simulink model "souk_single_pipeline_krm"  (R2021a)
settings: Solver=VariableStepAuto  StartTime=0.0  StopTime=10.0  RelTol=1e-3
undefined symbols (not defined in the file): datetime, emio_enet2_tsu_timer_cmp_val_0, posixtime, signal
libraries: xbsIndex_r4 x9043, casper_library_misc x75, casper_library_delays x33, casper_library_reorder x22, xps_library x11
(part 12 of 101)

== system souk_single_pipeline_krm/p0/synth_input_reorder ==
  note: split even / odd channels to separate streams,
      | since the downstream OS synth bank operates
      | on even and odd channels with independent
      | PSBs
  note: And now reverse back to multiple channels
      | per word
  sync : Inport
  din : Inport  Port=2
  rst : Inport  Port=3
  3 : Subsystem  AncestorBlock=casper_library_reorder/reorder  mask(reorder){map=reshape(transpose(reshape([0:2^(serial_chan_bits + parallel_samp_bits)-1], 2^parallel_samp_bits, [])), 2^(serial_chan_bits + parallel_samp_bits), []), n_bits=0, n_inputs=1, bram_latency=2, map_latency=1, fanout_latency=0, double_buffer=1, bram_map=off, software_controlled=off, use_control_fanout=on, hide_latency=on}
      mask prompts: map "Output Order:"; n_bits "Data width in"; n_inputs "Number of inputs"; bram_latency "BRAM Latency"; map_latency "Map Latency"; fanout_latency "Fanout latency"; double_buffer "Double Buffer"; bram_map "Use BlockRAM for Map"; software_controlled "Use runtime software control"; use_control_fanout "Control fanout of control to multiple iniputs"; hide_latency "EXPERIMENTAL: Hide control latency"
      mask init: same as souk_single_pipeline_krm/p0/chan_select/2
      settings: AttributesFormatString=order=2
      mask Help: eval('xlWeb(''http://casper.berkeley.edu/wiki/Reorder'')')
  Constant : xbsIndex_r4/Constant  Commented=on  const=1.0  gui_display_data_type=Boolean  arith_type=Boolean  n_bits=16  bin_pt=14  preci_type=Single  exp_width=8  frac_width=24  explicit_period=on  period=1  equ=P=C  opselect=C  inp2=PCIN>>17  opr=+  inp1=P  carry=CIN  dbl_ovrd=off  block_type=constant
  Constant4 : xbsIndex_r4/Constant  const=1.0  gui_display_data_type=Boolean  arith_type=Boolean  n_bits=16  bin_pt=14  preci_type=Single  exp_width=8  frac_width=24  explicit_period=on  period=1  equ=P=C  opselect=C  inp2=PCIN>>17  opr=+  inp1=P  carry=CIN  dbl_ovrd=off  block_type=constant
  Constant6 : xbsIndex_r4/Constant  Commented=on  const=2^15 - 1  gui_display_data_type=Fixed-point  arith_type=Unsigned  n_bits=15  bin_pt=0  preci_type=Single  exp_width=8  frac_width=24  explicit_period=on  period=1  equ=P=C  opselect=C  inp2=PCIN>>17  opr=+  inp1=P  carry=CIN  dbl_ovrd=off  block_type=constant
  Constant7 : xbsIndex_r4/Constant  Commented=on  const=1.0  gui_display_data_type=Boolean  arith_type=Boolean  n_bits=16  bin_pt=14  preci_type=Single  exp_width=8  frac_width=24  explicit_period=on  period=1  equ=P=C  opselect=C  inp2=PCIN>>17  opr=+  inp1=P  carry=CIN  dbl_ovrd=off  block_type=constant
  Counter : xbsIndex_r4/Counter  Commented=on  cnt_type=Free Running  cnt_to=Inf  operation=Up  start_count=0  cnt_by_val=1  arith_type=Unsigned  n_bits=15  bin_pt=0  load_pin=off  rst=on  en=off  explicit_period=on  period=1  use_behavioral_HDL=off  implementation=Fabric  dbl_ovrd=off  block_type=counter
  Delay1 : xbsIndex_r4/Delay  rst=off  infoeditControl=Selection of Reset will increase slice count due to use of real FFs and instead of SRLs  en=off  latency=0  reg_retiming=on  dbl_ovrd=off  block_type=delay
  Relational : xbsIndex_r4/Relational  Commented=on  mode=a=b  op_type=Bool  en=off  latency=0  dbl_ovrd=off  block_type=relational
  bus_convert : Subsystem  Commented=on  AncestorBlock=casper_library_bus/bus_convert  mask(bus_convert){n_bits_in=ones(8,1) * 18, bin_pt_in=17, cmplx=on, n_bits_out=16, bin_pt_out=15, quantization=0, overflow=0, csp_latency=0, of=off, misc=off}
      mask prompts: n_bits_in "input bit widths"; bin_pt_in "input binary points"; cmplx "input complex"; n_bits_out "output bit widths"; bin_pt_out "output binary points"; quantization "quantization strategy (Truncate=0, Round  (unbiased: +/- Inf)=1, Round (unbiased: Even Values)=2)"; overflow "overflow strategy (Wrap=0, Saturate=1, Flag as error=2)"; csp_latency "latency"; of "overflow indication"; misc "misc support"
      mask help: Convert components of busses
      mask init: same as souk_single_pipeline_krm/common/cordic_gen/bus_convert
  bus_convert1 : Subsystem  Commented=on  AncestorBlock=casper_library_bus/bus_convert  mask(bus_convert){n_bits_in=ones(8,1) * 18, bin_pt_in=17, cmplx=on, n_bits_out=16, bin_pt_out=15, quantization=0, overflow=0, csp_latency=0, of=off, misc=off}
      mask prompts: n_bits_in "input bit widths"; bin_pt_in "input binary points"; cmplx "input complex"; n_bits_out "output bit widths"; bin_pt_out "output binary points"; quantization "quantization strategy (Truncate=0, Round  (unbiased: +/- Inf)=1, Round (unbiased: Even Values)=2)"; overflow "overflow strategy (Wrap=0, Saturate=1, Flag as error=2)"; csp_latency "latency"; of "overflow indication"; misc "misc support"
      mask help: Convert components of busses
      mask init: same as souk_single_pipeline_krm/common/cordic_gen/bus_convert
  bus_convert2 : Subsystem  AncestorBlock=casper_library_bus/bus_convert  mask(bus_convert){n_bits_in=ones(4,1)*24, bin_pt_in=22, cmplx=on, n_bits_out=18, bin_pt_out=17, quantization=2, overflow=1, csp_latency=0, of=off, misc=off}
      mask prompts: n_bits_in "input bit widths"; bin_pt_in "input binary points"; cmplx "input complex"; n_bits_out "output bit widths"; bin_pt_out "output binary points"; quantization "quantization strategy (Truncate=0, Round  (unbiased: +/- Inf)=1, Round (unbiased: Even Values)=2)"; overflow "overflow strategy (Wrap=0, Saturate=1, Flag as error=2)"; csp_latency "latency"; of "overflow indication"; misc "misc support"
      mask help: Convert components of busses
      mask init: same as souk_single_pipeline_krm/common/cordic_gen/bus_convert
  bus_create : Subsystem  AncestorBlock=casper_library_flow_control/bus_create  mask(bus_create){inputNum=2^(parallel_chan_bits - parallel_samp_bits)}
      mask prompts: inputNum "Number of inputs:"
      mask init:
      | bus_create_init(gcb,...
      |     'inputNum', inputNum);
  bus_create1 : Subsystem  AncestorBlock=casper_library_flow_control/bus_create  mask(bus_create){inputNum=2^(parallel_samp_bits)}
      mask prompts: inputNum "Number of inputs:"
      mask init:
      | bus_create_init(gcb,...
      |     'inputNum', inputNum);
  bus_create2 : Subsystem  AncestorBlock=casper_library_flow_control/bus_create  mask(bus_create){inputNum=2^(parallel_samp_bits)}
      mask prompts: inputNum "Number of inputs:"
      mask init:
      | bus_create_init(gcb,...
      |     'inputNum', inputNum);
  bus_create3 : Subsystem  AncestorBlock=casper_library_flow_control/bus_create  mask(bus_create){inputNum=2^(parallel_samp_bits)}
      mask prompts: inputNum "Number of inputs:"
      mask init:
      | bus_create_init(gcb,...
      |     'inputNum', inputNum);
  bus_create4 : Subsystem  AncestorBlock=casper_library_flow_control/bus_create  mask(bus_create){inputNum=2^(parallel_samp_bits)}
      mask prompts: inputNum "Number of inputs:"
      mask init:
      | bus_create_init(gcb,...
      |     'inputNum', inputNum);
  bus_expand : Subsystem  AncestorBlock=casper_library_flow_control/bus_expand  mask(bus_expand){mode=divisions of equal size, outputNum=2, outputWidth=36 * 2^(parallel_chan_bits-1), outputBinaryPt=0, outputArithmeticType=0, show_format=off, outputToWorkspace=off, variablePrefix=out, outputToModelAsWell=on}
      mask prompts: outputNum "Number of outputs:"; outputWidth "Output width:"; outputBinaryPt "Output binary point position:"; outputArithmeticType "Output arithmetic type (ufix=0, fix=1, bool=2):"; show_format "Print format string?"; outputToWorkspace "Output to workspace?"; variablePrefix "Variable name prefix:"; outputToModelAsWell "Output to model as well?"
      mask help:
      | Expands a 'bus' made using a bus_create or Xilinx
      | concat block.
      | The input will be divided into the specified number
      | of outputs with the specified arithmetic types.
      | Divisions are made from most significant bit.
      mask init: same as souk_single_pipeline_krm/bus_expand
      settings: AttributesFormatString=2 outputs
      mask TypeOptions mode: divisions of equal size | divisions of arbitrary size
      mask Callback mode: %bus_expand_callback();
      mask Callback outputWidth: %bus_expand_callback();
      mask Callback outputToWorkspace: %bus_expand_callback();
  bus_expand1 : Subsystem  AncestorBlock=casper_library_flow_control/bus_expand  mask(bus_expand){mode=divisions of equal size, outputNum=2^parallel_samp_bits, outputWidth=18*2, outputBinaryPt=0, outputArithmeticType=0, show_format=off, outputToWorkspace=off, variablePrefix=out, outputToModelAsWell=on}
      mask prompts: outputNum "Number of outputs:"; outputWidth "Output width:"; outputBinaryPt "Output binary point position:"; outputArithmeticType "Output arithmetic type (ufix=0, fix=1, bool=2):"; show_format "Print format string?"; outputToWorkspace "Output to workspace?"; variablePrefix "Variable name prefix:"; outputToModelAsWell "Output to model as well?"
      mask help:
      | Expands a 'bus' made using a bus_create or Xilinx
      | concat block.
      | The input will be divided into the specified number
      | of outputs with the specified arithmetic types.
      | Divisions are made from most significant bit.
      mask init: same as souk_single_pipeline_krm/bus_expand
      settings: AttributesFormatString=4 outputs
      mask TypeOptions mode: divisions of equal size | divisions of arbitrary size
      mask Callback mode: %bus_expand_callback();
      mask Callback outputWidth: %bus_expand_callback();
      mask Callback outputToWorkspace: %bus_expand_callback();
  bus_expand2 : Subsystem  AncestorBlock=casper_library_flow_control/bus_expand  mask(bus_expand){mode=divisions of equal size, outputNum=2^parallel_samp_bits, outputWidth=18*2, outputBinaryPt=0, outputArithmeticType=0, show_format=off, outputToWorkspace=off, variablePrefix=out, outputToModelAsWell=on}
      mask prompts: outputNum "Number of outputs:"; outputWidth "Output width:"; outputBinaryPt "Output binary point position:"; outputArithmeticType "Output arithmetic type (ufix=0, fix=1, bool=2):"; show_format "Print format string?"; outputToWorkspace "Output to workspace?"; variablePrefix "Variable name prefix:"; outputToModelAsWell "Output to model as well?"
      mask help:
      | Expands a 'bus' made using a bus_create or Xilinx
      | concat block.
      | The input will be divided into the specified number
      | of outputs with the specified arithmetic types.
      | Divisions are made from most significant bit.
      mask init: same as souk_single_pipeline_krm/bus_expand
      settings: AttributesFormatString=4 outputs
      mask TypeOptions mode: divisions of equal size | divisions of arbitrary size
      mask Callback mode: %bus_expand_callback();
      mask Callback outputWidth: %bus_expand_callback();
      mask Callback outputToWorkspace: %bus_expand_callback();
  bus_expand3 : Subsystem  AncestorBlock=casper_library_flow_control/bus_expand  mask(bus_expand){mode=divisions of equal size, outputNum=2^parallel_samp_bits, outputWidth=18*2, outputBinaryPt=0, outputArithmeticType=0, show_format=off, outputToWorkspace=off, variablePrefix=out, outputToModelAsWell=on}
      mask prompts: outputNum "Number of outputs:"; outputWidth "Output width:"; outputBinaryPt "Output binary point position:"; outputArithmeticType "Output arithmetic type (ufix=0, fix=1, bool=2):"; show_format "Print format string?"; outputToWorkspace "Output to workspace?"; variablePrefix "Variable name prefix:"; outputToModelAsWell "Output to model as well?"
      mask help:
      | Expands a 'bus' made using a bus_create or Xilinx
      | concat block.
      | The input will be divided into the specified number
      | of outputs with the specified arithmetic types.
      | Divisions are made from most significant bit.
      mask init: same as souk_single_pipeline_krm/bus_expand
      settings: AttributesFormatString=4 outputs
      mask TypeOptions mode: divisions of equal size | divisions of arbitrary size
      mask Callback mode: %bus_expand_callback();
      mask Callback outputWidth: %bus_expand_callback();
      mask Callback outputToWorkspace: %bus_expand_callback();
  bus_expand4 : Subsystem  AncestorBlock=casper_library_flow_control/bus_expand  mask(bus_expand){mode=divisions of equal size, outputNum=2^parallel_samp_bits, outputWidth=18*2, outputBinaryPt=0, outputArithmeticType=0, show_format=off, outputToWorkspace=off, variablePrefix=out, outputToModelAsWell=on}
      mask prompts: outputNum "Number of outputs:"; outputWidth "Output width:"; outputBinaryPt "Output binary point position:"; outputArithmeticType "Output arithmetic type (ufix=0, fix=1, bool=2):"; show_format "Print format string?"; outputToWorkspace "Output to workspace?"; variablePrefix "Variable name prefix:"; outputToModelAsWell "Output to model as well?"
      mask help:
      | Expands a 'bus' made using a bus_create or Xilinx
      | concat block.
      | The input will be divided into the specified number
      | of outputs with the specified arithmetic types.
      | Divisions are made from most significant bit.
      mask init: same as souk_single_pipeline_krm/bus_expand
      settings: AttributesFormatString=4 outputs
      mask TypeOptions mode: divisions of equal size | divisions of arbitrary size
      mask Callback mode: %bus_expand_callback();
      mask Callback outputWidth: %bus_expand_callback();
      mask Callback outputToWorkspace: %bus_expand_callback();
  map0 : Subsystem  mask{vec_len_bits=11, ram_latency=2, sample_width=18, n_samples=2^parallel_samp_bits, add_latency=2}
      mask prompts: vec_len_bits "Vector length (2^?)"; ram_latency "Ram Latency"; sample_width "data width per sample"; n_samples "Number of samples per word"; add_latency "Adder latency"
  map1 : Subsystem  mask{vec_len_bits=11, ram_latency=2, sample_width=18, n_samples=2^parallel_samp_bits, add_latency=2}
      mask prompts: vec_len_bits "Vector length (2^?)"; ram_latency "Ram Latency"; sample_width "data width per sample"; n_samples "Number of samples per word"; add_latency "Adder latency"
  map2 : Subsystem  mask{vec_len_bits=11, ram_latency=2, sample_width=18, n_samples=2^parallel_samp_bits, add_latency=2}
      mask prompts: vec_len_bits "Vector length (2^?)"; ram_latency "Ram Latency"; sample_width "data width per sample"; n_samples "Number of samples per word"; add_latency "Adder latency"
  map3 : Subsystem  mask{vec_len_bits=11, ram_latency=2, sample_width=18, n_samples=2^parallel_samp_bits, add_latency=2}
      mask prompts: vec_len_bits "Vector length (2^?)"; ram_latency "Ram Latency"; sample_width "data width per sample"; n_samples "Number of samples per word"; add_latency "Adder latency"
  munge1 : Subsystem  AncestorBlock=casper_library_flow_control/munge  mask(munge){divisions=2^parallel_chan_bits, div_size=ones(2^parallel_chan_bits, 1) * 36, order=reshape(transpose(reshape([0:2^parallel_chan_bits - 1], 2, [])), 1, []), arith_type_out=Unsigned, bin_pt_out=0}
      mask prompts: divisions "Number of divisions"; div_size "Division size (bits)"; order "Division packing order"; arith_type_out "Output arithmetic type"; bin_pt_out "Output binary point"
      mask help: Splits an input bus into the specified number of divisions and then recombines them in the order specified (most significant division = 0,least = number divisions-1)
      mask init:
      | munge_init(gcb, ...
      |     'divisions', divisions, ...
      |     'div_size', div_size, ...
      |     'order', order, ...
      |     'arith_type_out', arith_type_out, ...
      |     'bin_pt_out', bin_pt_out);
      settings: AttributesFormatString=|
      | split:[36;36;36;36;36;36;36;36;36;36;36;36;36;36;36;36]
      | join:[0 2 4 6 8 10 12 14 1 3 5 7 9 11 13 15]
      | Unsigned [576,0]
      mask TypeOptions arith_type_out: Unsigned | Signed  (2's comp) | Floating-point
  snapshot0 : Subsystem  Tag=casper:snapshot  Commented=on  AncestorBlock=casper_library_scopes/snapshot  mask(snapshot){storage=bram, dram_dimm=2, dram_clock=250, nsamples=13, data_width=256, offset=off, circap=off, value=off, ext_arm=off, ext_circ=off, provide_outputs=on, use_dsp48=off}
      mask prompts: storage "Storage medium"; dram_dimm "DRAM dimm"; dram_clock "DRAM clock rate"; nsamples "Number of Samples (2^?)"; data_width "Data width"; offset "Start delay support"; circap "Circular capture support"; value "Extra value capture support"; ext_arm "External arm support"; ext_circ "External circular capture support"; provide_outputs "Provide outputs"; use_dsp48 "Use DSP48s to implement counters"
      mask help:
      | Standard snap block, but with the following optional extras;
      |  1) Optionally delay the fabric trigger by a user-specified number of valids.
      |  2) Capture continuously after a trigger until a stop pulse is received. Data is captured into BRAM continuously, with old data being overwritten until a stop command is received. Then stop capturing when memory is filled. This enables you to get some data before and some data after the stop pulse. Use the 'tr_en_cnt' register to determine where you are in your vector. 'Addr' register's MSb now indicates 'busy capturing'.
      |  3) Optionally capture a value on an input port to a register at the same time as the first data sample.
      |  4) Implement counters using DSP48Es to save resources.
      mask init: same as souk_single_pipeline_krm/p0/acc0/snapshot
      settings: AttributesFormatString=|
      | 256 wide, 8192 deep
      | debugID: 87241941
      mask TypeOptions storage: bram | dram
      mask Callback storage: snapshot_callback();
      mask TypeOptions dram_dimm: 1 | 2 | 3 | 4
      mask TypeOptions dram_clock: 200 | 250 | 266 | 300 | 333
      mask TypeOptions data_width: 8 | 16 | 32 | 64 | 128 | 256 | 512 | 1024
  snapshot1 : Subsystem  Tag=casper:snapshot  Commented=on  AncestorBlock=casper_library_scopes/snapshot  mask(snapshot){storage=bram, dram_dimm=2, dram_clock=250, nsamples=13, data_width=256, offset=off, circap=off, value=off, ext_arm=off, ext_circ=off, provide_outputs=on, use_dsp48=off}
      mask prompts: storage "Storage medium"; dram_dimm "DRAM dimm"; dram_clock "DRAM clock rate"; nsamples "Number of Samples (2^?)"; data_width "Data width"; offset "Start delay support"; circap "Circular capture support"; value "Extra value capture support"; ext_arm "External arm support"; ext_circ "External circular capture support"; provide_outputs "Provide outputs"; use_dsp48 "Use DSP48s to implement counters"
      mask help:
      | Standard snap block, but with the following optional extras;
      |  1) Optionally delay the fabric trigger by a user-specified number of valids.
      |  2) Capture continuously after a trigger until a stop pulse is received. Data is captured into BRAM continuously, with old data being overwritten until a stop command is received. Then stop capturing when memory is filled. This enables you to get some data before and some data after the stop pulse. Use the 'tr_en_cnt' register to determine where you are in your vector. 'Addr' register's MSb now indicates 'busy capturing'.
      |  3) Optionally capture a value on an input port to a register at the same time as the first data sample.
      |  4) Implement counters using DSP48Es to save resources.
      mask init: same as souk_single_pipeline_krm/p0/acc0/snapshot
      settings: AttributesFormatString=|
      | 256 wide, 8192 deep
      | debugID: 87241941
      mask TypeOptions storage: bram | dram
      mask Callback storage: snapshot_callback();
      mask TypeOptions dram_dimm: 1 | 2 | 3 | 4
      mask TypeOptions dram_clock: 200 | 250 | 266 | 300 | 333
      mask TypeOptions data_width: 8 | 16 | 32 | 64 | 128 | 256 | 512 | 1024
  square_transposer1 : Subsystem  AncestorBlock=casper_library_reorder/square_transposer  mask(square_transposer){n_inputs=parallel_samp_bits, async=off}
      mask prompts: n_inputs "Number of inputs (2^?):"; async "Aynchronus operation"
      mask init:
      | square_transposer_init(gcb,...
      |     'n_inputs', n_inputs, ...
      |     'async', async);
      settings: AttributesFormatString=n_inputs=2
      mask Help: eval('xlWeb(''http://casper.berkeley.edu/wiki/Square_transposer'')')
  square_transposer2 : Subsystem  AncestorBlock=casper_library_reorder/square_transposer  mask(square_transposer){n_inputs=parallel_samp_bits, async=off}
      mask prompts: n_inputs "Number of inputs (2^?):"; async "Aynchronus operation"
      mask init:
      | square_transposer_init(gcb,...
      |     'n_inputs', n_inputs, ...
      |     'async', async);
      settings: AttributesFormatString=n_inputs=2
      mask Help: eval('xlWeb(''http://casper.berkeley.edu/wiki/Square_transposer'')')
  square_transposer3 : Subsystem  AncestorBlock=casper_library_reorder/square_transposer  mask(square_transposer){n_inputs=parallel_samp_bits, async=off}
      mask prompts: n_inputs "Number of inputs (2^?):"; async "Aynchronus operation"
      mask init:
      | square_transposer_init(gcb,...
      |     'n_inputs', n_inputs, ...
      |     'async', async);
      settings: AttributesFormatString=n_inputs=2
      mask Help: eval('xlWeb(''http://casper.berkeley.edu/wiki/Square_transposer'')')
  square_transposer4 : Subsystem  AncestorBlock=casper_library_reorder/square_transposer  mask(square_transposer){n_inputs=parallel_samp_bits, async=off}
      mask prompts: n_inputs "Number of inputs (2^?):"; async "Aynchronus operation"
      mask init:
      | square_transposer_init(gcb,...
      |     'n_inputs', n_inputs, ...
      |     'async', async);
      settings: AttributesFormatString=n_inputs=2
      mask Help: eval('xlWeb(''http://casper.berkeley.edu/wiki/Square_transposer'')')
  sync_out : Outport  VectorParamsAs1DForOutWhenUnconnected=off
  dout0 : Outport  Port=2  VectorParamsAs1DForOutWhenUnconnected=off
  dout1 : Outport  Port=3  VectorParamsAs1DForOutWhenUnconnected=off
  wires:
  bus_create4/1(bus_out) -> bus_create/4(in4)
  bus_create1/1(bus_out) -> bus_create/1(in1)
  bus_create3/1(bus_out) -> bus_create/3(in3)
  bus_create2/1(bus_out) -> bus_create/2(in2)
  map3/1(sync_out) -> square_transposer4/1(sync)
  map3/2(dout) -> bus_expand4/1(bus_in)
  square_transposer4/2(out0) -> bus_create4/1(in1)
  square_transposer4/3(out1) -> bus_create4/2(in2)
  square_transposer4/4(out2) -> bus_create4/3(in3)
  square_transposer4/5(out3) -> bus_create4/4(in4)
  bus_expand4/1(msb_out4) -> square_transposer4/2(in0)
  bus_expand4/2(out3) -> square_transposer4/3(in1)
  bus_expand4/3(out2) -> square_transposer4/4(in2)
  bus_expand4/4(lsb_out1) -> square_transposer4/5(in3)
  bus_expand3/4(lsb_out1) -> square_transposer3/5(in3)
  bus_expand3/3(out2) -> square_transposer3/4(in2)
  bus_expand3/2(out3) -> square_transposer3/3(in1)
  bus_expand3/1(msb_out4) -> square_transposer3/2(in0)
  square_transposer3/5(out3) -> bus_create3/4(in4)
  square_transposer3/4(out2) -> bus_create3/3(in3)
  square_transposer3/3(out1) -> bus_create3/2(in2)
  square_transposer3/2(out0) -> bus_create3/1(in1)
  map2/2(dout) -> bus_expand3/1(bus_in)
  map2/1(sync_out) -> square_transposer3/1(sync)
  map1/1(sync_out) -> square_transposer2/1(sync)
  map1/2(dout) -> bus_expand2/1(bus_in)
  square_transposer2/2(out0) -> bus_create2/1(in1)
  square_transposer2/3(out1) -> bus_create2/2(in2)
  square_transposer2/4(out2) -> bus_create2/3(in3)
  square_transposer2/5(out3) -> bus_create2/4(in4)
  bus_expand2/1(msb_out4) -> square_transposer2/2(in0)
  bus_expand2/2(out3) -> square_transposer2/3(in1)
  bus_expand2/3(out2) -> square_transposer2/4(in2)
  bus_expand2/4(lsb_out1) -> square_transposer2/5(in3)
  bus_create/1(bus_out) -> 3/3(din0)
  munge1/1(dout) -> bus_expand/1(bus_in)
  bus_expand/1(msb_out2) -> bus_convert/1(din), dout0/1
  bus_expand/2(lsb_out1) -> bus_convert1/1(din), dout1/1
  3/3(dout0) -> munge1/1(din)
  3/1(sync_out) -> Counter/1, sync_out/1
  bus_expand1/4(lsb_out1) -> square_transposer1/5(in3)
  bus_expand1/3(out2) -> square_transposer1/4(in2)
  bus_expand1/2(out3) -> square_transposer1/3(in1)
  bus_expand1/1(msb_out4) -> square_transposer1/2(in0)
  sync/1 -> Delay1/1
  din/1 -> bus_convert2/1(din)
  square_transposer1/5(out3) -> bus_create1/4(in4)
  square_transposer1/4(out2) -> bus_create1/3(in3)
  square_transposer1/3(out1) -> bus_create1/2(in2)
  square_transposer1/2(out0) -> bus_create1/1(in1)
  map0/2(dout) -> bus_expand1/1(bus_in)
  map0/1(sync_out) -> square_transposer1/1(sync)
  Constant4/1 -> 3/2(en)
  square_transposer1/1(sync_out) -> 3/1(sync)
  Delay1/1 -> map1/1(sync), map3/1(sync), map2/1(sync), map0/1(sync)
  bus_convert2/1(dout) -> map0/2(din), map1/2(din), map3/2(din), map2/2(din)
  bus_convert/1(dout) -> snapshot0/1(din)
  Constant/1 -> snapshot0/2(we)
  Counter/1 -> Relational/1
  Constant6/1 -> Relational/2
  Relational/1 -> snapshot1/3(trig), snapshot0/3(trig)
  Constant7/1 -> snapshot1/2(we)
  bus_convert1/1(dout) -> snapshot1/1(din)
  rst/1 -> map0/3(rst), map1/3(rst), map3/3(rst), map2/3(rst)

== system souk_single_pipeline_krm/p0/synth_input_reorder1 ==
  note: And now reverse back to multiple channels
      | per word
  sync : Inport
  din : Inport  Port=2
  1 : Subsystem  AncestorBlock=casper_library_reorder/reorder  mask(reorder){map=reshape(transpose(reshape([0:2^(serial_chan_bits + parallel_chan_bits)-1], 2^parallel_chan_bits, [])), 2^(serial_chan_bits + parallel_chan_bits), []), n_bits=0, n_inputs=1, bram_latency=3, map_latency=1, fanout_latency=0, double_buffer=0, bram_map=off, software_controlled=off}
      mask prompts: map "Output Order:"; n_bits "Data width in"; n_inputs "Number of inputs"; bram_latency "BRAM Latency"; map_latency "Map Latency"; fanout_latency "Fanout latency"; double_buffer "Double Buffer"; bram_map "Use BlockRAM for Map"; software_controlled "Use runtime software control"
      mask init:
      | reorder_init(gcb, ...
      |     'map', map, ...
      |     'n_bits', n_bits, ...
      |     'n_inputs', n_inputs, ...
      |     'bram_latency', bram_latency, ...
      |     'map_latency', map_latency, ...
      |     'fanout_latency', fanout_latency, ...
      |     'double_buffer', double_buffer, ...
      |     'bram_map', bram_map, ...
      |     'software_controlled', software_controlled);
      settings: AttributesFormatString=order=11
      mask Help: eval('xlWeb(''http://casper.berkeley.edu/wiki/Reorder'')')
  3 : Subsystem  AncestorBlock=casper_library_reorder/reorder  mask(reorder){map=reshape(transpose(reshape([0:2^(serial_chan_bits + parallel_chan_bits)-1], 2^parallel_chan_bits, [])), 2^(serial_chan_bits + parallel_chan_bits), []), n_bits=0, n_inputs=1, bram_latency=3, map_latency=1, fanout_latency=0, double_buffer=0, bram_map=off, software_controlled=off}
      mask prompts: map "Output Order:"; n_bits "Data width in"; n_inputs "Number of inputs"; bram_latency "BRAM Latency"; map_latency "Map Latency"; fanout_latency "Fanout latency"; double_buffer "Double Buffer"; bram_map "Use BlockRAM for Map"; software_controlled "Use runtime software control"
      mask init: same as souk_single_pipeline_krm/p0/synth_input_reorder1/1
      settings: AttributesFormatString=order=11
      mask Help: eval('xlWeb(''http://casper.berkeley.edu/wiki/Reorder'')')
  Constant{,2,6..11} (8 alike) : xbsIndex_r4/Constant  const=0  gui_display_data_type=Fixed-point  arith_type=Unsigned  n_bits=36  bin_pt=0  preci_type=Single  exp_width=8  frac_width=24  explicit_period=on  period=1  equ=P=C  opselect=C  inp2=PCIN>>17  opr=+  inp1=P  carry=CIN  dbl_ovrd=off  block_type=constant
  Constant{1,3..5} (4 alike) : xbsIndex_r4/Constant  const=1.0  gui_display_data_type=Boolean  arith_type=Boolean  n_bits=16  bin_pt=14  preci_type=Single  exp_width=8  frac_width=24  explicit_period=on  period=1  equ=P=C  opselect=C  inp2=PCIN>>17  opr=+  inp1=P  carry=CIN  dbl_ovrd=off  block_type=constant
  bus_create1 : Subsystem  AncestorBlock=casper_library_flow_control/bus_create  mask(bus_create){inputNum=2^(parallel_chan_bits+1)}
      mask prompts: inputNum "Number of inputs:"
      mask init:
      | bus_create_init(gcb,...
      |     'inputNum', inputNum);
  bus_create2 : Subsystem  AncestorBlock=casper_library_flow_control/bus_create  mask(bus_create){inputNum=2^(parallel_chan_bits+1)}
      mask prompts: inputNum "Number of inputs:"
      mask init:
      | bus_create_init(gcb,...
      |     'inputNum', inputNum);
  bus_expand1 : Subsystem  AncestorBlock=casper_library_flow_control/bus_expand  mask(bus_expand){mode=divisions of equal size, outputNum=2^parallel_chan_bits, outputWidth=18*2, outputBinaryPt=0, outputArithmeticType=0, show_format=off, outputToWorkspace=off, variablePrefix=out, outputToModelAsWell=on}
      mask prompts: outputNum "Number of outputs:"; outputWidth "Output width:"; outputBinaryPt "Output binary point position:"; outputArithmeticType "Output arithmetic type (ufix=0, fix=1, bool=2):"; show_format "Print format string?"; outputToWorkspace "Output to workspace?"; variablePrefix "Variable name prefix:"; outputToModelAsWell "Output to model as well?"
      mask help:
      | Expands a 'bus' made using a bus_create or Xilinx
      | concat block.
      | The input will be divided into the specified number
      | of outputs with the specified arithmetic types.
      | Divisions are made from most significant bit.
      mask init: same as souk_single_pipeline_krm/bus_expand
      settings: AttributesFormatString=4 outputs
      mask TypeOptions mode: divisions of equal size | divisions of arbitrary size
      mask Callback mode: %bus_expand_callback();
      mask Callback outputWidth: %bus_expand_callback();
      mask Callback outputToWorkspace: %bus_expand_callback();
  bus_expand2 : Subsystem  AncestorBlock=casper_library_flow_control/bus_expand  mask(bus_expand){mode=divisions of equal size, outputNum=2^parallel_chan_bits, outputWidth=18*2, outputBinaryPt=0, outputArithmeticType=0, show_format=off, outputToWorkspace=off, variablePrefix=out, outputToModelAsWell=on}
      mask prompts: outputNum "Number of outputs:"; outputWidth "Output width:"; outputBinaryPt "Output binary point position:"; outputArithmeticType "Output arithmetic type (ufix=0, fix=1, bool=2):"; show_format "Print format string?"; outputToWorkspace "Output to workspace?"; variablePrefix "Variable name prefix:"; outputToModelAsWell "Output to model as well?"
      mask help:
      | Expands a 'bus' made using a bus_create or Xilinx
      | concat block.
      | The input will be divided into the specified number
      | of outputs with the specified arithmetic types.
      | Divisions are made from most significant bit.
      mask init: same as souk_single_pipeline_krm/bus_expand
      settings: AttributesFormatString=4 outputs
      mask TypeOptions mode: divisions of equal size | divisions of arbitrary size
      mask Callback mode: %bus_expand_callback();
      mask Callback outputWidth: %bus_expand_callback();
      mask Callback outputToWorkspace: %bus_expand_callback();
  map0 : Subsystem  AncestorBlock=casper_library_reorder/reorder  mask(reorder){map=[2^(serial_chan_bits + parallel_chan_bits+1)-1:-1:0], n_bits=0, n_inputs=1, bram_latency=3, map_latency=1, fanout_latency=0, double_buffer=1, bram_map=off, software_controlled=on}
      mask prompts: map "Output Order:"; n_bits "Data width in"; n_inputs "Number of inputs"; bram_latency "BRAM Latency"; map_latency "Map Latency"; fanout_latency "Fanout latency"; double_buffer "Double Buffer"; bram_map "Use BlockRAM for Map"; software_controlled "Use runtime software control"
      mask init: same as souk_single_pipeline_krm/p0/synth_input_reorder1/1
      settings: AttributesFormatString=order=2
      mask Help: eval('xlWeb(''http://casper.berkeley.edu/wiki/Reorder'')')
  map1 : Subsystem  AncestorBlock=casper_library_reorder/reorder  mask(reorder){map=[2^(serial_chan_bits + parallel_chan_bits+1)-1:-1:0], n_bits=0, n_inputs=1, bram_latency=3, map_latency=1, fanout_latency=0, double_buffer=1, bram_map=off, software_controlled=on}
      mask prompts: map "Output Order:"; n_bits "Data width in"; n_inputs "Number of inputs"; bram_latency "BRAM Latency"; map_latency "Map Latency"; fanout_latency "Fanout latency"; double_buffer "Double Buffer"; bram_map "Use BlockRAM for Map"; software_controlled "Use runtime software control"
      mask init: same as souk_single_pipeline_krm/p0/synth_input_reorder1/1
      settings: AttributesFormatString=order=2
      mask Help: eval('xlWeb(''http://casper.berkeley.edu/wiki/Reorder'')')
  square_transposer1 : Subsystem  AncestorBlock=casper_library_reorder/square_transposer  mask(square_transposer){n_inputs=parallel_chan_bits+1, async=off}
      mask prompts: n_inputs "Number of inputs (2^?):"; async "Aynchronus operation"
      mask init:
      | square_transposer_init(gcb,...
      |     'n_inputs', n_inputs, ...
      |     'async', async);
      settings: AttributesFormatString=n_inputs=3
      mask Help: eval('xlWeb(''http://casper.berkeley.edu/wiki/Square_transposer'')')
  square_transposer2 : Subsystem  AncestorBlock=casper_library_reorder/square_transposer  mask(square_transposer){n_inputs=parallel_chan_bits+1, async=off}
      mask prompts: n_inputs "Number of inputs (2^?):"; async "Aynchronus operation"
      mask init:
      | square_transposer_init(gcb,...
      |     'n_inputs', n_inputs, ...
      |     'async', async);
      settings: AttributesFormatString=n_inputs=3
      mask Help: eval('xlWeb(''http://casper.berkeley.edu/wiki/Square_transposer'')')
  sync_out : Outport  VectorParamsAs1DForOutWhenUnconnected=off
  dout0 : Outport  Port=2  VectorParamsAs1DForOutWhenUnconnected=off
  dout1 : Outport  Port=3  VectorParamsAs1DForOutWhenUnconnected=off
  wires:
  square_transposer2/8(out6) -> bus_create2/7(in7)
  Constant10/1 -> square_transposer2/8(in6)
  Constant11/1 -> square_transposer2/9(in7)
  Constant8/1 -> square_transposer2/6(in4)
  Constant9/1 -> square_transposer2/7(in5)
  Constant7/1 -> square_transposer1/9(in7)
  Constant6/1 -> square_transposer1/8(in6)
  Constant2/1 -> square_transposer1/7(in5)
  Constant/1 -> square_transposer1/6(in4)
  bus_expand2/4(lsb_out1) -> square_transposer2/5(in3)
  bus_expand2/3(out2) -> square_transposer2/4(in2)
  bus_expand2/2(out3) -> square_transposer2/3(in1)
  bus_expand2/1(msb_out4) -> square_transposer2/2(in0)
  bus_expand1/4(lsb_out1) -> square_transposer1/5(in3)
  bus_expand1/3(out2) -> square_transposer1/4(in2)
  bus_expand1/2(out3) -> square_transposer1/3(in1)
  bus_expand1/1(msb_out4) -> square_transposer1/2(in0)
  1/3(dout0) -> dout1/1
  Constant5/1 -> map1/2(en)
  bus_create2/1(bus_out) -> 1/3(din0)
  square_transposer2/1(sync_out) -> 1/1(sync)
  Constant3/1 -> 1/2(en)
  map1/1(sync_out) -> square_transposer2/1(sync)
  map1/3(dout0) -> bus_expand2/1(bus_in)
  square_transposer2/2(out0) -> bus_create2/1(in1)
  square_transposer2/3(out1) -> bus_create2/2(in2)
  square_transposer2/4(out2) -> bus_create2/3(in3)
  square_transposer2/5(out3) -> bus_create2/4(in4)
  ? -> ?
  square_transposer2/6(out4) -> bus_create2/5(in5)
  square_transposer2/7(out5) -> bus_create2/6(in6)
  square_transposer2/9(out7) -> bus_create2/8(in8)
  3/1(sync_out) -> sync_out/1
  3/3(dout0) -> dout0/1
  sync/1 -> map0/1(sync), map1/1(sync)
  din/1 -> map0/3(din0), map1/3(din0)
  Constant1/1 -> map0/2(en)
  square_transposer1/9(out7) -> bus_create1/8(in8)
  square_transposer1/8(out6) -> bus_create1/7(in7)
  square_transposer1/7(out5) -> bus_create1/6(in6)
  square_transposer1/6(out4) -> bus_create1/5(in5)
  square_transposer1/5(out3) -> bus_create1/4(in4)
  square_transposer1/4(out2) -> bus_create1/3(in3)
  square_transposer1/3(out1) -> bus_create1/2(in2)
  square_transposer1/2(out0) -> bus_create1/1(in1)
  map0/3(dout0) -> bus_expand1/1(bus_in)
  map0/1(sync_out) -> square_transposer1/1(sync)
  Constant4/1 -> 3/2(en)
  square_transposer1/1(sync_out) -> 3/1(sync)
  bus_create1/1(bus_out) -> 3/3(din0)
